simulink model "ControlModule"  (R2019b)
settings: Solver=VariableStepAuto  StartTime=0.0  StopTime=10.0  RelTol=1e-3
settings Model: Creator=loker  LastModifiedBy=loker

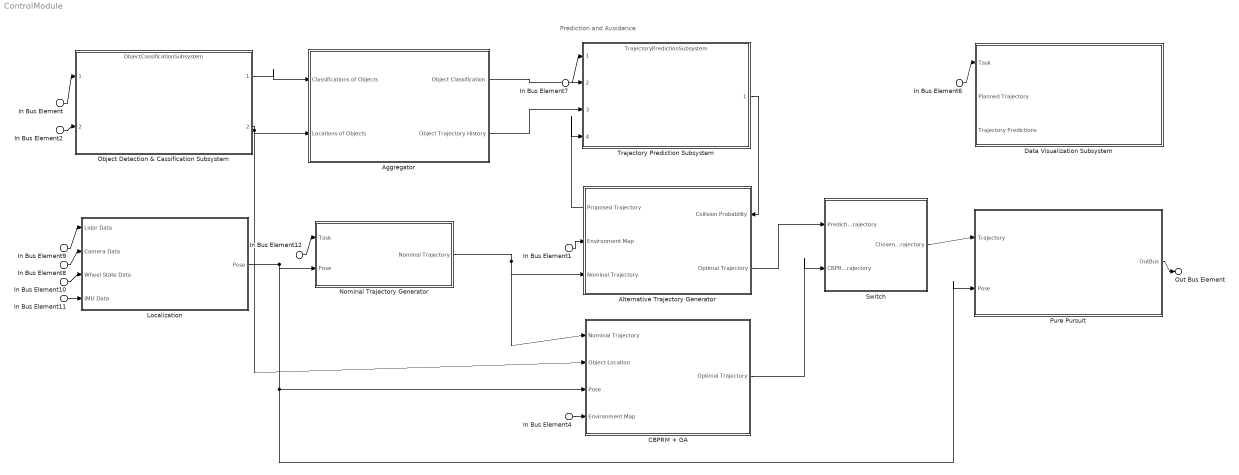
== system ControlModule ==
  note: Prediction and Avoidence
  In Bus Element7 : Inport  PortName=Trajectory Dictionary
  In Bus Element : Inport  Port=2  PortName=Camera Data
  In Bus Element8 : Inport  Port=2  PortName=Camera Data
  In Bus Element9 : Inport  Port=3  PortName=Lidar Data
  In Bus Element2 : Inport  Port=3  PortName=Lidar Data
  In Bus Element11 : Inport  Port=4  PortName=IMU Data
  In Bus Element10 : Inport  Port=5  PortName=Wheel State Data
  In Bus Element4 : Inport  Port=6  PortName=Environment Map
  In Bus Element1 : Inport  Port=6  PortName=Environment Map
  In Bus Element6 : Inport  Port=7  PortName=Task
  In Bus Element12 : Inport  Port=7  PortName=Task
  Aggregator : Subsystem
      settings: PortSchema="{\"entries\":[{\"content\":{\"headerSize\":26,\"margin\":15,\"minimumSpacing\":25,\"sides\":[{\"content\":{\"connectorIds\":[\"In1\",\"In2\"]},\"type\":\"ConnectorPlacement.EquallySpacedRectSide\",\"uuid\":\"e969fe28-f86a-4134-aa48-ac5e7d1e883d\"},{\"content\":{\"connectorIds\":[\"Out1\",\"Out2\"],\"side\":\"RIGHT\"},\"type\":\"ConnectorPlacement.EquallySpacedRectSide\",\"uuid\":\"60451ad4-053f-474e-b513-91540490c4d6\"},{\"content\":{\"connectorIds\":[],\"side\":\"TOP\"},\"type\":\"ConnectorPlacement.EquallySpacedRectSide\",\"uuid\":\"8c0a71ec-10d4-4c65-a834-1a5cda01dd40\"}]},\"type\":\"ConnectorPlacement.EquallySpacedConnector\",\"uuid\":\"9b9a34e7-bab3-4005-850a-799bc8dbb258\"}],\"packageUris\":[\"http://schema.mathworks.com/mf0/Connector/19700101\"],\"version\":\"1.0\"}"
  Alternative Trajectory Generator : Subsystem
      settings: PortSchema="{\"entries\":[{\"content\":{\"headerSize\":26,\"margin\":15,\"minimumSpacing\":25,\"sides\":[{\"content\":{\"connectorIds\":[\"Out1\",\"In2\",\"In1\"]},\"type\":\"ConnectorPlacement.EquallySpacedRectSide\",\"uuid\":\"e969fe28-f86a-4134-aa48-ac5e7d1e883d\"},{\"content\":{\"connectorIds\":[\"In3\",\"Out2\"],\"side\":\"RIGHT\"},\"type\":\"ConnectorPlacement.EquallySpacedRectSide\",\"uuid\":\"60451ad4-053f-474e-b513-91540490c4d6\"},{\"content\":{\"connectorIds\":[],\"side\":\"TOP\"},\"type\":\"ConnectorPlacement.EquallySpacedRectSide\",\"uuid\":\"8c0a71ec-10d4-4c65-a834-1a5cda01dd40\"}]},\"type\":\"ConnectorPlacement.EquallySpacedConnector\",\"uuid\":\"9b9a34e7-bab3-4005-850a-799bc8dbb258\"}],\"packageUris\":[\"http://schema.mathworks.com/mf0/Connector/19700101\"],\"version\":\"1.0\"}"
  CBPRM + GA : Subsystem
      settings: PortSchema="{\"entries\":[{\"content\":{\"headerSize\":26,\"margin\":15,\"minimumSpacing\":25,\"sides\":[{\"content\":{\"connectorIds\":[\"In1\",\"In2\",\"In3\",\"In4\"]},\"type\":\"ConnectorPlacement.EquallySpacedRectSide\",\"uuid\":\"e969fe28-f86a-4134-aa48-ac5e7d1e883d\"},{\"content\":{\"connectorIds\":[\"Out1\"],\"side\":\"RIGHT\"},\"type\":\"ConnectorPlacement.EquallySpacedRectSide\",\"uuid\":\"60451ad4-053f-474e-b513-91540490c4d6\"},{\"content\":{\"connectorIds\":[],\"side\":\"TOP\"},\"type\":\"ConnectorPlacement.EquallySpacedRectSide\",\"uuid\":\"8c0a71ec-10d4-4c65-a834-1a5cda01dd40\"}]},\"type\":\"ConnectorPlacement.EquallySpacedConnector\",\"uuid\":\"9b9a34e7-bab3-4005-850a-799bc8dbb258\"}],\"packageUris\":[\"http://schema.mathworks.com/mf0/Connector/19700101\"],\"version\":\"1.0\"}"
  Data Visualization Subsystem : Subsystem
      settings: PortSchema="{\"entries\":[{\"content\":{\"headerSize\":26,\"margin\":15,\"minimumSpacing\":25,\"sides\":[{\"content\":{\"connectorIds\":[\"In1\",\"In2\",\"In3\"]},\"type\":\"ConnectorPlacement.EquallySpacedRectSide\",\"uuid\":\"9c658e47-9141-4b09-899d-e7d6eeef288e\"},{\"content\":{\"connectorIds\":[],\"side\":\"RIGHT\"},\"type\":\"ConnectorPlacement.EquallySpacedRectSide\",\"uuid\":\"7a582264-0565-42d4-adb3-e560ad597e55\"},{\"content\":{\"connectorIds\":[],\"side\":\"TOP\"},\"type\":\"ConnectorPlacement.EquallySpacedRectSide\",\"uuid\":\"701b4c6c-e203-4bd7-b8b7-cb8feb01699c\"}]},\"type\":\"ConnectorPlacement.EquallySpacedConnector\",\"uuid\":\"2059a5e9-c0d5-4fb6-87cf-b1bfdc666ab8\"}],\"packageUris\":[\"http://schema.mathworks.com/mf0/Connector/19700101\"],\"version\":\"1.0\"}"
  Localization : Subsystem
      settings: PortSchema="{\"entries\":[{\"content\":{\"headerSize\":26,\"margin\":15,\"minimumSpacing\":25,\"sides\":[{\"content\":{\"connectorIds\":[\"In1\",\"In2\",\"In3\",\"In4\"]},\"type\":\"ConnectorPlacement.EquallySpacedRectSide\",\"uuid\":\"e969fe28-f86a-4134-aa48-ac5e7d1e883d\"},{\"content\":{\"connectorIds\":[\"Out1\"],\"side\":\"RIGHT\"},\"type\":\"ConnectorPlacement.EquallySpacedRectSide\",\"uuid\":\"60451ad4-053f-474e-b513-91540490c4d6\"},{\"content\":{\"connectorIds\":[],\"side\":\"TOP\"},\"type\":\"ConnectorPlacement.EquallySpacedRectSide\",\"uuid\":\"8c0a71ec-10d4-4c65-a834-1a5cda01dd40\"}]},\"type\":\"ConnectorPlacement.EquallySpacedConnector\",\"uuid\":\"9b9a34e7-bab3-4005-850a-799bc8dbb258\"}],\"packageUris\":[\"http://schema.mathworks.com/mf0/Connector/19700101\"],\"version\":\"1.0\"}"
  Nominal Trajectory Generator : Subsystem
      settings: PortSchema="{\"entries\":[{\"content\":{\"headerSize\":26,\"margin\":15,\"minimumSpacing\":25,\"sides\":[{\"content\":{\"connectorIds\":[\"In1\",\"In2\"]},\"type\":\"ConnectorPlacement.EquallySpacedRectSide\",\"uuid\":\"e969fe28-f86a-4134-aa48-ac5e7d1e883d\"},{\"content\":{\"connectorIds\":[\"Out1\"],\"side\":\"RIGHT\"},\"type\":\"ConnectorPlacement.EquallySpacedRectSide\",\"uuid\":\"60451ad4-053f-474e-b513-91540490c4d6\"},{\"content\":{\"connectorIds\":[],\"side\":\"TOP\"},\"type\":\"ConnectorPlacement.EquallySpacedRectSide\",\"uuid\":\"8c0a71ec-10d4-4c65-a834-1a5cda01dd40\"}]},\"type\":\"ConnectorPlacement.EquallySpacedConnector\",\"uuid\":\"9b9a34e7-bab3-4005-850a-799bc8dbb258\"}],\"packageUris\":[\"http://schema.mathworks.com/mf0/Connector/19700101\"],\"version\":\"1.0\"}"
  Object Detection & Cassification Subsystem : ModelReference  ModelNameDialog=ObjectCassificationSubsystem  SimulationMode=Normal  ModelReferenceVersion=1.2
      settings: PortSchema="{\"entries\":[{\"content\":{\"headerSize\":38,\"margin\":15,\"minimumSpacing\":25,\"sides\":[{\"content\":{\"connectorIds\":[\"In1\",\"In2\"]},\"type\":\"ConnectorPlacement.EquallySpacedRectSide\",\"uuid\":\"9c658e47-9141-4b09-899d-e7d6eeef288e\"},{\"content\":{\"connectorIds\":[\"Out1\",\"Out2\"],\"side\":\"RIGHT\"},\"type\":\"ConnectorPlacement.EquallySpacedRectSide\",\"uuid\":\"7a582264-0565-42d4-adb3-e560ad597e55\"},{\"content\":{\"connectorIds\":[],\"side\":\"TOP\"},\"type\":\"ConnectorPlacement.EquallySpacedRectSide\",\"uuid\":\"701b4c6c-e203-4bd7-b8b7-cb8feb01699c\"}]},\"type\":\"ConnectorPlacement.EquallySpacedConnector\",\"uuid\":\"2059a5e9-c0d5-4fb6-87cf-b1bfdc666ab8\"}],\"packageUris\":[\"http://schema.mathworks.com/mf0/Connector/19700101\"],\"version\":\"1.0\"}"
  Pure Pursuit : Subsystem
      settings: PortSchema="{\"entries\":[{\"content\":{\"headerSize\":26,\"margin\":15,\"minimumSpacing\":25,\"sides\":[{\"content\":{\"connectorIds\":[\"In1\",\"In2\"]},\"type\":\"ConnectorPlacement.EquallySpacedRectSide\",\"uuid\":\"e969fe28-f86a-4134-aa48-ac5e7d1e883d\"},{\"content\":{\"connectorIds\":[\"Out1\"],\"side\":\"RIGHT\"},\"type\":\"ConnectorPlacement.EquallySpacedRectSide\",\"uuid\":\"60451ad4-053f-474e-b513-91540490c4d6\"},{\"content\":{\"connectorIds\":[],\"side\":\"TOP\"},\"type\":\"ConnectorPlacement.EquallySpacedRectSide\",\"uuid\":\"8c0a71ec-10d4-4c65-a834-1a5cda01dd40\"}]},\"type\":\"ConnectorPlacement.EquallySpacedConnector\",\"uuid\":\"9b9a34e7-bab3-4005-850a-799bc8dbb258\"}],\"packageUris\":[\"http://schema.mathworks.com/mf0/Connector/19700101\"],\"version\":\"1.0\"}"
  Switch : Subsystem
      settings: PortSchema="{\"entries\":[{\"content\":{\"headerSize\":26,\"margin\":15,\"minimumSpacing\":25,\"sides\":[{\"content\":{\"connectorIds\":[\"In1\",\"In2\"]},\"type\":\"ConnectorPlacement.EquallySpacedRectSide\",\"uuid\":\"e969fe28-f86a-4134-aa48-ac5e7d1e883d\"},{\"content\":{\"connectorIds\":[\"Out1\"],\"side\":\"RIGHT\"},\"type\":\"ConnectorPlacement.EquallySpacedRectSide\",\"uuid\":\"60451ad4-053f-474e-b513-91540490c4d6\"},{\"content\":{\"connectorIds\":[],\"side\":\"TOP\"},\"type\":\"ConnectorPlacement.EquallySpacedRectSide\",\"uuid\":\"8c0a71ec-10d4-4c65-a834-1a5cda01dd40\"}]},\"type\":\"ConnectorPlacement.EquallySpacedConnector\",\"uuid\":\"9b9a34e7-bab3-4005-850a-799bc8dbb258\"}],\"packageUris\":[\"http://schema.mathworks.com/mf0/Connector/19700101\"],\"version\":\"1.0\"}"
  Trajectory Prediction Subsystem : ModelReference  ModelNameDialog=TrajectoryPredictionSubsystem  SimulationMode=Normal  ModelReferenceVersion=1.4
      settings: PortSchema="{\"entries\":[{\"content\":{\"headerSize\":38,\"margin\":15,\"minimumSpacing\":25,\"sides\":[{\"content\":{\"connectorIds\":[\"In1\",\"In2\",\"In3\",\"In4\"]},\"type\":\"ConnectorPlacement.EquallySpacedRectSide\",\"uuid\":\"9c658e47-9141-4b09-899d-e7d6eeef288e\"},{\"content\":{\"connectorIds\":[\"Out1\"],\"side\":\"RIGHT\"},\"type\":\"ConnectorPlacement.EquallySpacedRectSide\",\"uuid\":\"7a582264-0565-42d4-adb3-e560ad597e55\"},{\"content\":{\"connectorIds\":[],\"side\":\"TOP\"},\"type\":\"ConnectorPlacement.EquallySpacedRectSide\",\"uuid\":\"701b4c6c-e203-4bd7-b8b7-cb8feb01699c\"}]},\"type\":\"ConnectorPlacement.EquallySpacedConnector\",\"uuid\":\"2059a5e9-c0d5-4fb6-87cf-b1bfdc666ab8\"}],\"packageUris\":[\"http://schema.mathworks.com/mf0/Connector/19700101\"],\"version\":\"1.0\"}"
  Out Bus Element : Outport  PortName=Desired Wheel State
  wires:
  In Bus Element/1 -> Object Detection & Cassification Subsystem/1
  In Bus Element6/1 -> Data Visualization Subsystem/1(Task)
  In Bus Element7/1 -> Trajectory Prediction Subsystem/1
  In Bus Element8/1 -> Localization/2(Camera Data)
  In Bus Element9/1 -> Localization/1(Lidar Data)
  In Bus Element10/1 -> Localization/3(Wheel State Data)
  In Bus Element11/1 -> Localization/4(IMU Data)
  In Bus Element12/1 -> Nominal Trajectory Generator/1(Task)
  Localization/1(Pose) -> Pure Pursuit/2(Pose), CBPRM + GA/3(Pose), Nominal Trajectory Generator/2(Pose)
  Trajectory Prediction Subsystem/1 -> Alternative Trajectory Generator/3(Collision Probability)
  Nominal Trajectory Generator/1(Nominal Trajectory) -> CBPRM + GA/1(Nominal Trajectory), Alternative Trajectory Generator/1(Nominal Trajectory)
  Pure Pursuit/1(OutBus) -> Out Bus Element/1
  In Bus Element4/1 -> CBPRM + GA/4(Environment Map)
  In Bus Element1/1 -> Alternative Trajectory Generator/2(Environment Map)
  Alternative Trajectory Generator/2(Optimal Trajectory) -> Switch/1(Predictive Trajectory)
  CBPRM + GA/1(Optimal Trajectory) -> Switch/2(CBPRM Trajectory)
  Switch/1(Chosen Trajectory) -> Pure Pursuit/1(Trajectory)
  Object Detection & Cassification Subsystem/2 -> Aggregator/2(Locations of Objects), CBPRM + GA/2(Object Location)
  Object Detection & Cassification Subsystem/1 -> Aggregator/1(Classifications of Objects)
  Alternative Trajectory Generator/1(Proposed Trajectory) -> Trajectory Prediction Subsystem/4
  Aggregator/2(Object Trajectory History) -> Trajectory Prediction Subsystem/3
  Aggregator/1(Object Classification) -> Trajectory Prediction Subsystem/2
  In Bus Element2/1 -> Object Detection & Cassification Subsystem/2

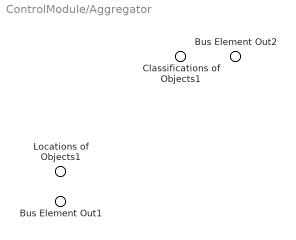
== system ControlModule/Aggregator ==
  Classifications of Objects1 : Inport  PortName=Classifications of Objects
  Locations of Objects1 : Inport  Port=2  PortName=Locations of Objects
  Bus Element Out2 : Outport  PortName=Object Classification
  Bus Element Out1 : Outport  Port=2  PortName=Object Trajectory History

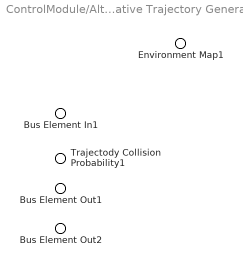
== system ControlModule/Alternative Trajectory Generator ==
  Bus Element In1 : Inport  PortName=Nominal Trajectory
  Environment Map1 : Inport  Port=2  PortName=Environment Map
  Trajectody Collision Probability1 : Inport  Port=3  PortName=Collision Probability
  Bus Element Out1 : Outport  PortName=Proposed Trajectory
  Bus Element Out2 : Outport  Port=2  PortName=Optimal Trajectory

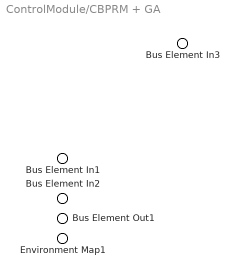
== system ControlModule/CBPRM + GA ==
  Bus Element In3 : Inport  PortName=Nominal Trajectory
  Bus Element In1 : Inport  Port=2  PortName=Object Location
  Bus Element In2 : Inport  Port=3  PortName=Pose
  Environment Map1 : Inport  Port=4  PortName=Environment Map
  Bus Element Out1 : Outport  PortName=Optimal Trajectory

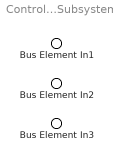
== system ControlModule/Data Visualization Subsystem ==
  Bus Element In1 : Inport  PortName=Task
  Bus Element In2 : Inport  Port=2  PortName=Planned Trajectory
  Bus Element In3 : Inport  Port=3  PortName=Trajectory Predictions

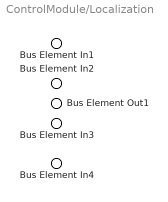
== system ControlModule/Localization ==
  Bus Element In1 : Inport  PortName=Lidar Data
  Bus Element In2 : Inport  Port=2  PortName=Camera Data
  Bus Element In3 : Inport  Port=3  PortName=Wheel State Data
  Bus Element In4 : Inport  Port=4  PortName=IMU Data
  Bus Element Out1 : Outport  PortName=Pose

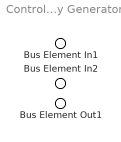
== system ControlModule/Nominal Trajectory Generator ==
  Bus Element In1 : Inport  PortName=Task
  Bus Element In2 : Inport  Port=2  PortName=Pose
  Bus Element Out1 : Outport  PortName=Nominal Trajectory

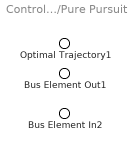
== system ControlModule/Pure Pursuit ==
  Optimal Trajectory1 : Inport  PortName=Trajectory
  Bus Element In2 : Inport  Port=2  PortName=Pose
  Bus Element Out1 : Outport  PortName=OutBus

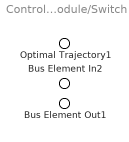
== system ControlModule/Switch ==
  Optimal Trajectory1 : Inport  PortName=Predictive Trajectory
  Bus Element In2 : Inport  Port=2  PortName=CBPRM Trajectory
  Bus Element Out1 : Outport  PortName=Chosen Trajectory
